simulink library "ssc_Probes_2014a_org"  (Simulink 10.0)
settings: Solver=ode45  StartTime=0.0  StopTime=10.0  RelTol=1e-3  EnableMultiTasking=on
libraries: fl_lib x50, nesl_utility x49, pe_lib x9
(part 2 of 3)

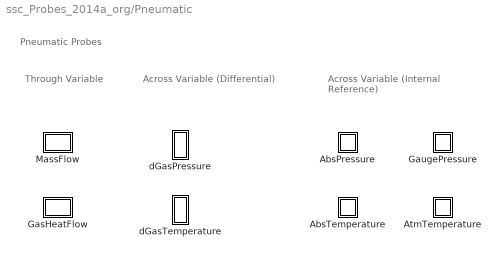
== system ssc_Probes_2014a_org/Pneumatic ==
  note: Pneumatic Probes
  note: Across Variable
      | (Internal Reference)
  note: Through
      | Variable
  note: Across Variable
      | (Differential)
  AbsPressure : Subsystem  Description=Simscape Probe  InitFcn=|
      | unit=get_param([gcb '/PS-S'],'Unit');                                              
      | set_param(gcb, 'AttributesFormatString', strcat('[', unit,']'));
      mask help: Simscape Probe
      settings: CopyFcn=|
      | if strcmp(get_param(gcb, 'LinkStatus'),'implicit') == 0;
      | set_param(gcb,'LinkStatus','inactive');
      | set_param(gcb,'LinkStatus','none');
      | end
      | set_param([gcb '/Goto'],'GotoTag', [get(gcbh,'name')]);
      | set_param([gcb '/From'],'GotoTag', [get(gcbh,'name')]);
      | h = get_param([gcb, '/PS-S'], 'PortHandles');
      | set(h.Outport(1), 'SignalNameFromLabel', [get(gcbh,'name')])
      | clear h;
      settings: NameChangeFcn=|
      | set_param([gcb '/Goto'],'GotoTag', [get(gcbh,'name')]);
      | set_param([gcb '/From'],'GotoTag', [get(gcbh,'name')]);
      | h = get_param([gcb, '/PS-S'], 'PortHandles');
      | set(h.Outport(1), 'SignalNameFromLabel', [get(gcbh,'name')])
      | clear h;
      settings: OpenFcn=|
      | if exist('logsout', 'var')
      |   vname = get(gcbh,'name');
      |   fHandle = findall(0,'Tag',vname);
      |   if isempty(fHandle)
      |   figure('Tag',vname);
      |   end;
      |   figure(findobj('Tag',vname));
      |   plot(logsout.getElement([gcb, '/PS-S'], '-blockpath').Values)
      |   title(get(gcbh,'name'));
      |   ylabel(['Pressure (' get_param([gcb '/PS-S'],'Unit') ')'] );
      | end
      mask Display: port_label('LConn', 1,'P');
  AbsTemperature : Subsystem  Description=Simscape Probe  InitFcn=|
      | unit=get_param([gcb '/PS-S'],'Unit');                                              
      | set_param(gcb, 'AttributesFormatString', strcat('[', unit,']'));
      mask help: Simscape Probe
      settings: CopyFcn=|
      | if strcmp(get_param(gcb, 'LinkStatus'),'implicit') == 0;
      | set_param(gcb,'LinkStatus','inactive');
      | set_param(gcb,'LinkStatus','none');
      | end
      | set_param([gcb '/Goto'],'GotoTag', [get(gcbh,'name')]);
      | set_param([gcb '/From'],'GotoTag', [get(gcbh,'name')]);
      | h = get_param([gcb, '/PS-S'], 'PortHandles');
      | set(h.Outport(1), 'SignalNameFromLabel', [get(gcbh,'name')])
      | clear h;
      settings: NameChangeFcn=|
      | set_param([gcb '/Goto'],'GotoTag', [get(gcbh,'name')]);
      | set_param([gcb '/From'],'GotoTag', [get(gcbh,'name')]);
      | h = get_param([gcb, '/PS-S'], 'PortHandles');
      | set(h.Outport(1), 'SignalNameFromLabel', [get(gcbh,'name')])
      | clear h;
      settings: OpenFcn=|
      | if exist('logsout', 'var')
      |   vname = get(gcbh,'name');
      |   fHandle = findall(0,'Tag',vname);
      |   if isempty(fHandle)
      |   figure('Tag',vname);
      |   end;
      |   figure(findobj('Tag',vname));
      |   plot(logsout.getElement([gcb, '/PS-S'], '-blockpath').Values)
      |   title(get(gcbh,'name'));
      |   ylabel(['Temperature (' get_param([gcb '/PS-S'],'Unit') ')'] );
      | end
      mask Display: port_label('LConn', 1,'T');
  AtmTemperature : Subsystem  Description=Simscape Probe  InitFcn=|
      | unit=get_param([gcb '/PS-S'],'Unit');                                              
      | set_param(gcb, 'AttributesFormatString', strcat('[', unit,']'));
      mask help: Simscape Probe
      settings: CopyFcn=|
      | if strcmp(get_param(gcb, 'LinkStatus'),'implicit') == 0;
      | set_param(gcb,'LinkStatus','inactive');
      | set_param(gcb,'LinkStatus','none');
      | end
      | set_param([gcb '/Goto'],'GotoTag', [get(gcbh,'name')]);
      | set_param([gcb '/From'],'GotoTag', [get(gcbh,'name')]);
      | h = get_param([gcb, '/PS-S'], 'PortHandles');
      | set(h.Outport(1), 'SignalNameFromLabel', [get(gcbh,'name')])
      | clear h;
      settings: NameChangeFcn=|
      | set_param([gcb '/Goto'],'GotoTag', [get(gcbh,'name')]);
      | set_param([gcb '/From'],'GotoTag', [get(gcbh,'name')]);
      | h = get_param([gcb, '/PS-S'], 'PortHandles');
      | set(h.Outport(1), 'SignalNameFromLabel', [get(gcbh,'name')])
      | clear h;
      settings: OpenFcn=|
      | if exist('logsout', 'var')
      |   vname = get(gcbh,'name');
      |   fHandle = findall(0,'Tag',vname);
      |   if isempty(fHandle)
      |   figure('Tag',vname);
      |   end;
      |   figure(findobj('Tag',vname));
      |   plot(logsout.getElement([gcb, '/PS-S'], '-blockpath').Values)
      |   title(get(gcbh,'name'));
      |   ylabel(['Temperature (' get_param([gcb '/PS-S'],'Unit') ')'] );
      | end
      mask Display: port_label('LConn', 1,'T');
  GasHeatFlow : Subsystem  Description=Simscape Probe  InitFcn=|
      | unit=get_param([gcb '/PS-S'],'Unit');                                              
      | set_param(gcb, 'AttributesFormatString', strcat('[', unit,']'));
      mask help: Simscape Probe
      settings: CopyFcn=|
      | if strcmp(get_param(gcb, 'LinkStatus'),'implicit') == 0;
      | set_param(gcb,'LinkStatus','inactive');
      | set_param(gcb,'LinkStatus','none');
      | end
      | set_param([gcb '/Goto'],'GotoTag', [get(gcbh,'name')]);
      | set_param([gcb '/From'],'GotoTag', [get(gcbh,'name')]);
      | h = get_param([gcb, '/PS-S'], 'PortHandles');
      | set(h.Outport(1), 'SignalNameFromLabel', [get(gcbh,'name')])
      | clear h;
      settings: NameChangeFcn=|
      | set_param([gcb '/Goto'],'GotoTag', [get(gcbh,'name')]);
      | set_param([gcb '/From'],'GotoTag', [get(gcbh,'name')]);
      | h = get_param([gcb, '/PS-S'], 'PortHandles');
      | set(h.Outport(1), 'SignalNameFromLabel', [get(gcbh,'name')])
      | clear h;
      settings: OpenFcn=|
      | if exist('logsout', 'var')
      |   vname = get(gcbh,'name');
      |   fHandle = findall(0,'Tag',vname);
      |   if isempty(fHandle)
      |   figure('Tag',vname);
      |   end;
      |   figure(findobj('Tag',vname));
      |   plot(logsout.getElement([gcb, '/PS-S'], '-blockpath').Values)
      |   title(get(gcbh,'name'));
      |   ylabel(['Heat Flow (' get_param([gcb '/PS-S'],'Unit') ')'] );
      | end
      mask Display:
      | patch([0.5 1 0.5], [0.25 .5 0.75],[0.7 0.7 0.7])
      | plot([0,0.5],[0.5,0.5]);
  GaugePressure : Subsystem  Description=Simscape Probe  InitFcn=|
      | unit=get_param([gcb '/PS-S'],'Unit');                                              
      | set_param(gcb, 'AttributesFormatString', strcat('[', unit,']'));
      mask help: Simscape Probe
      settings: CopyFcn=|
      | if strcmp(get_param(gcb, 'LinkStatus'),'implicit') == 0;
      | set_param(gcb,'LinkStatus','inactive');
      | set_param(gcb,'LinkStatus','none');
      | end
      | set_param([gcb '/Goto'],'GotoTag', [get(gcbh,'name')]);
      | set_param([gcb '/From'],'GotoTag', [get(gcbh,'name')]);
      | h = get_param([gcb, '/PS-S'], 'PortHandles');
      | set(h.Outport(1), 'SignalNameFromLabel', [get(gcbh,'name')])
      | clear h;
      settings: NameChangeFcn=|
      | set_param([gcb '/Goto'],'GotoTag', [get(gcbh,'name')]);
      | set_param([gcb '/From'],'GotoTag', [get(gcbh,'name')]);
      | h = get_param([gcb, '/PS-S'], 'PortHandles');
      | set(h.Outport(1), 'SignalNameFromLabel', [get(gcbh,'name')])
      | clear h;
      settings: OpenFcn=|
      | if exist('logsout', 'var')
      |   vname = get(gcbh,'name');
      |   fHandle = findall(0,'Tag',vname);
      |   if isempty(fHandle)
      |   figure('Tag',vname);
      |   end;
      |   figure(findobj('Tag',vname));
      |   plot(logsout.getElement([gcb, '/PS-S'], '-blockpath').Values)
      |   title(get(gcbh,'name'));
      |   ylabel(['Pressure (' get_param([gcb '/PS-S'],'Unit') ')'] );
      | end
      mask Display: port_label('LConn', 1,'P');
  MassFlow : Subsystem  Description=Simscape Probe  InitFcn=|
      | unit=get_param([gcb '/PS-S'],'Unit');                                              
      | set_param(gcb, 'AttributesFormatString', strcat('[', unit,']'));
      mask help: Simscape Probe
      settings: CopyFcn=|
      | if strcmp(get_param(gcb, 'LinkStatus'),'implicit') == 0;
      | set_param(gcb,'LinkStatus','inactive');
      | set_param(gcb,'LinkStatus','none');
      | end
      | set_param([gcb '/Goto'],'GotoTag', [get(gcbh,'name')]);
      | set_param([gcb '/From'],'GotoTag', [get(gcbh,'name')]);
      | h = get_param([gcb, '/PS-S'], 'PortHandles');
      | set(h.Outport(1), 'SignalNameFromLabel', [get(gcbh,'name')])
      | clear h;
      settings: NameChangeFcn=|
      | set_param([gcb '/Goto'],'GotoTag', [get(gcbh,'name')]);
      | set_param([gcb '/From'],'GotoTag', [get(gcbh,'name')]);
      | h = get_param([gcb, '/PS-S'], 'PortHandles');
      | set(h.Outport(1), 'SignalNameFromLabel', [get(gcbh,'name')])
      | clear h;
      settings: OpenFcn=|
      | if exist('logsout', 'var')
      |   vname = get(gcbh,'name');
      |   fHandle = findall(0,'Tag',vname);
      |   if isempty(fHandle)
      |   figure('Tag',vname);
      |   end;
      |   figure(findobj('Tag',vname));
      |   plot(logsout.getElement([gcb, '/PS-S'], '-blockpath').Values)
      |   title(get(gcbh,'name'));
      |   ylabel(['Mass Flow (' get_param([gcb '/PS-S'],'Unit') ')'] );
      | end
      mask Display:
      | patch([0.5 1 0.5], [0.25 .5 0.75],[0.7 0.7 0.7])
      | plot([0,0.5],[0.5,0.5]);
  dGasPressure : Subsystem  Description=Simscape Probe  InitFcn=|
      | unit=get_param([gcb '/PS-S'],'Unit');                                              
      | set_param(gcb, 'AttributesFormatString', strcat('[', unit,']'));
      mask help: Simscape Probe
      settings: CopyFcn=|
      | if strcmp(get_param(gcb, 'LinkStatus'),'implicit') == 0;
      | set_param(gcb,'LinkStatus','inactive');
      | set_param(gcb,'LinkStatus','none');
      | end
      | set_param([gcb '/Goto'],'GotoTag', [get(gcbh,'name')]);
      | set_param([gcb '/From'],'GotoTag', [get(gcbh,'name')]);
      | h = get_param([gcb, '/PS-S'], 'PortHandles');
      | set(h.Outport(1), 'SignalNameFromLabel', [get(gcbh,'name')])
      | clear h;
      settings: NameChangeFcn=|
      | set_param([gcb '/Goto'],'GotoTag', [get(gcbh,'name')]);
      | set_param([gcb '/From'],'GotoTag', [get(gcbh,'name')]);
      | h = get_param([gcb, '/PS-S'], 'PortHandles');
      | set(h.Outport(1), 'SignalNameFromLabel', [get(gcbh,'name')])
      | clear h;
      settings: OpenFcn=|
      | if exist('logsout', 'var')
      |   vname = get(gcbh,'name');
      |   fHandle = findall(0,'Tag',vname);
      |   if isempty(fHandle)
      |   figure('Tag',vname);
      |   end;
      |   figure(findobj('Tag',vname));
      |   plot(logsout.getElement([gcb, '/PS-S'], '-blockpath').Values)
      |   title(get(gcbh,'name'));
      |   ylabel(['Pressure (' get_param([gcb '/PS-S'],'Unit') ')'] );
      | end
      mask Display:
      | port_label('RConn', 1,'-');
      | port_label('LConn', 1,'+');
  dGasTemperature : Subsystem  Description=Simscape Probe  InitFcn=|
      | unit=get_param([gcb '/PS-S'],'Unit');                                              
      | set_param(gcb, 'AttributesFormatString', strcat('[', unit,']'));
      mask help: Simscape Probe
      settings: CopyFcn=|
      | if strcmp(get_param(gcb, 'LinkStatus'),'implicit') == 0;
      | set_param(gcb,'LinkStatus','inactive');
      | set_param(gcb,'LinkStatus','none');
      | end
      | set_param([gcb '/Goto'],'GotoTag', [get(gcbh,'name')]);
      | set_param([gcb '/From'],'GotoTag', [get(gcbh,'name')]);
      | h = get_param([gcb, '/PS-S'], 'PortHandles');
      | set(h.Outport(1), 'SignalNameFromLabel', [get(gcbh,'name')])
      | clear h;
      settings: NameChangeFcn=|
      | set_param([gcb '/Goto'],'GotoTag', [get(gcbh,'name')]);
      | set_param([gcb '/From'],'GotoTag', [get(gcbh,'name')]);
      | h = get_param([gcb, '/PS-S'], 'PortHandles');
      | set(h.Outport(1), 'SignalNameFromLabel', [get(gcbh,'name')])
      | clear h;
      settings: OpenFcn=|
      | if exist('logsout', 'var')
      |   vname = get(gcbh,'name');
      |   fHandle = findall(0,'Tag',vname);
      |   if isempty(fHandle)
      |   figure('Tag',vname);
      |   end;
      |   figure(findobj('Tag',vname));
      |   plot(logsout.getElement([gcb, '/PS-S'], '-blockpath').Values)
      |   title(get(gcbh,'name'));
      |   ylabel(['Temperature (' get_param([gcb '/PS-S'],'Unit') ')'] );
      | end
      mask Display:
      | port_label('RConn', 1,'-');
      | port_label('LConn', 1,'+');

== system ssc_Probes_2014a_org/Thermal ==
  note: Thermal Probes
  note: Across Variable
      | (Internal Reference)
  note: Through
      | Variable
  note: Across Variable
      | (Differential)
  HeatFlow : Subsystem  Description=Simscape Probe  InitFcn=|
      | unit=get_param([gcb '/PS-S'],'Unit');                                              
      | set_param(gcb, 'AttributesFormatString', strcat('[', unit,']'));
      mask help: Simscape Probe
      settings: CopyFcn=|
      | if strcmp(get_param(gcb, 'LinkStatus'),'implicit') == 0;
      | set_param(gcb,'LinkStatus','inactive');
      | set_param(gcb,'LinkStatus','none');
      | end
      | set_param([gcb '/Goto'],'GotoTag', [get(gcbh,'name')]);
      | set_param([gcb '/From'],'GotoTag', [get(gcbh,'name')]);
      | h = get_param([gcb, '/PS-S'], 'PortHandles');
      | set(h.Outport(1), 'SignalNameFromLabel', [get(gcbh,'name')])
      | clear h;
      settings: NameChangeFcn=|
      | set_param([gcb '/Goto'],'GotoTag', [get(gcbh,'name')]);
      | set_param([gcb '/From'],'GotoTag', [get(gcbh,'name')]);
      | h = get_param([gcb, '/PS-S'], 'PortHandles');
      | set(h.Outport(1), 'SignalNameFromLabel', [get(gcbh,'name')])
      | clear h;
      settings: OpenFcn=|
      | if exist('logsout', 'var')
      |   vname = get(gcbh,'name');
      |   fHandle = findall(0,'Tag',vname);
      |   if isempty(fHandle)
      |   figure('Tag',vname);
      |   end;
      |   figure(findobj('Tag',vname));
      |   plot(logsout.getElement([gcb, '/PS-S'], '-blockpath').Values)
      |   title(get(gcbh,'name'));
      |   ylabel(['Heat Flow (' get_param([gcb '/PS-S'],'Unit') ')'] );
      | end
      mask Display:
      | patch([0.5 1 0.5], [0.25 .5 0.75],[0.7 0.7 0.7])
      | plot([0,0.5],[0.5,0.5]);
  Temperature : Subsystem  Description=Simscape Probe  InitFcn=|
      | unit=get_param([gcb '/PS-S'],'Unit');                                              
      | set_param(gcb, 'AttributesFormatString', strcat('[', unit,']'));
      mask help: Simscape Probe
      settings: CopyFcn=|
      | if strcmp(get_param(gcb, 'LinkStatus'),'implicit') == 0;
      | set_param(gcb,'LinkStatus','inactive');
      | set_param(gcb,'LinkStatus','none');
      | end
      | set_param([gcb '/Goto'],'GotoTag', [get(gcbh,'name')]);
      | set_param([gcb '/From'],'GotoTag', [get(gcbh,'name')]);
      | h = get_param([gcb, '/PS-S'], 'PortHandles');
      | set(h.Outport(1), 'SignalNameFromLabel', [get(gcbh,'name')])
      | clear h;
      settings: NameChangeFcn=|
      | set_param([gcb '/Goto'],'GotoTag', [get(gcbh,'name')]);
      | set_param([gcb '/From'],'GotoTag', [get(gcbh,'name')]);
      | h = get_param([gcb, '/PS-S'], 'PortHandles');
      | set(h.Outport(1), 'SignalNameFromLabel', [get(gcbh,'name')])
      | clear h;
      settings: OpenFcn=|
      | if exist('logsout', 'var')
      |   vname = get(gcbh,'name');
      |   fHandle = findall(0,'Tag',vname);
      |   if isempty(fHandle)
      |   figure('Tag',vname);
      |   end;
      |   figure(findobj('Tag',vname));
      |   plot(logsout.getElement([gcb, '/PS-S'], '-blockpath').Values)
      |   title(get(gcbh,'name'));
      |   ylabel(['Temperature (' get_param([gcb '/PS-S'],'Unit') ')'] );
      | end
      mask Display: port_label('LConn', 1,'T');
  dTemperature : Subsystem  Description=Simscape Probe  InitFcn=|
      | unit=get_param([gcb '/PS-S'],'Unit');                                              
      | set_param(gcb, 'AttributesFormatString', strcat('[', unit,']'));
      mask help: Simscape Probe
      settings: CopyFcn=|
      | if strcmp(get_param(gcb, 'LinkStatus'),'implicit') == 0;
      | set_param(gcb,'LinkStatus','inactive');
      | set_param(gcb,'LinkStatus','none');
      | end
      | set_param([gcb '/Goto'],'GotoTag', [get(gcbh,'name')]);
      | set_param([gcb '/From'],'GotoTag', [get(gcbh,'name')]);
      | h = get_param([gcb, '/PS-S'], 'PortHandles');
      | set(h.Outport(1), 'SignalNameFromLabel', [get(gcbh,'name')])
      | clear h;
      settings: NameChangeFcn=|
      | set_param([gcb '/Goto'],'GotoTag', [get(gcbh,'name')]);
      | set_param([gcb '/From'],'GotoTag', [get(gcbh,'name')]);
      | h = get_param([gcb, '/PS-S'], 'PortHandles');
      | set(h.Outport(1), 'SignalNameFromLabel', [get(gcbh,'name')])
      | clear h;
      settings: OpenFcn=|
      | if exist('logsout', 'var')
      |   vname = get(gcbh,'name');
      |   fHandle = findall(0,'Tag',vname);
      |   if isempty(fHandle)
      |   figure('Tag',vname);
      |   end;
      |   figure(findobj('Tag',vname));
      |   plot(logsout.getElement([gcb, '/PS-S'], '-blockpath').Values)
      |   title(get(gcbh,'name'));
      |   ylabel(['Temperature (' get_param([gcb '/PS-S'],'Unit') ')'] );
      | end
      mask Display:
      | port_label('RConn', 1,'-');
      | port_label('LConn', 1,'+');

== system ssc_Probes_2014a_org/ThermalLiquid ==
  note: Across Variable
      | (Differential)
  note: Through
      | Variable
  note: Across Variable
      | (Internal Reference)
  note: Thermal Probes
  AbsPressure_TL : Subsystem  Description=Simscape Probe  InitFcn=|
      | unit=get_param([gcb '/PS-S'],'Unit');                                              
      | set_param(gcb, 'AttributesFormatString', strcat('[', unit,']'));
      mask help: Simscape Probe
      settings: CopyFcn=|
      | if strcmp(get_param(gcb, 'LinkStatus'),'implicit') == 0;
      | set_param(gcb,'LinkStatus','inactive');
      | set_param(gcb,'LinkStatus','none');
      | end
      | set_param([gcb '/Goto'],'GotoTag', [get(gcbh,'name')]);
      | set_param([gcb '/From'],'GotoTag', [get(gcbh,'name')]);
      | h = get_param([gcb, '/PS-S'], 'PortHandles');
      | set(h.Outport(1), 'SignalNameFromLabel', [get(gcbh,'name')])
      | clear h;
      settings: NameChangeFcn=|
      | set_param([gcb '/Goto'],'GotoTag', [get(gcbh,'name')]);
      | set_param([gcb '/From'],'GotoTag', [get(gcbh,'name')]);
      | h = get_param([gcb, '/PS-S'], 'PortHandles');
      | set(h.Outport(1), 'SignalNameFromLabel', [get(gcbh,'name')])
      | clear h;
      settings: OpenFcn=|
      | if exist('logsout', 'var')
      |   vname = get(gcbh,'name');
      |   fHandle = findall(0,'Tag',vname);
      |   if isempty(fHandle)
      |   figure('Tag',vname);
      |   end;
      |   figure(findobj('Tag',vname));
      |   plot(logsout.getElement([gcb, '/PS-S'], '-blockpath').Values)
      |   title(get(gcbh,'name'));
      |   ylabel(['Pressure (' get_param([gcb '/PS-S'],'Unit') ')'] );
      | end
      mask Display: port_label('LConn', 1,'P');
  AbsTemperature_TL : Subsystem  Description=Simscape Probe  InitFcn=|
      | unit=get_param([gcb '/PS-S'],'Unit');                                              
      | set_param(gcb, 'AttributesFormatString', strcat('[', unit,']'));
      mask help: Simscape Probe
      settings: CopyFcn=|
      | if strcmp(get_param(gcb, 'LinkStatus'),'implicit') == 0;
      | set_param(gcb,'LinkStatus','inactive');
      | set_param(gcb,'LinkStatus','none');
      | end
      | set_param([gcb '/Goto'],'GotoTag', [get(gcbh,'name')]);
      | set_param([gcb '/From'],'GotoTag', [get(gcbh,'name')]);
      | h = get_param([gcb, '/PS-S'], 'PortHandles');
      | set(h.Outport(1), 'SignalNameFromLabel', [get(gcbh,'name')])
      | clear h;
      settings: NameChangeFcn=|
      | set_param([gcb '/Goto'],'GotoTag', [get(gcbh,'name')]);
      | set_param([gcb '/From'],'GotoTag', [get(gcbh,'name')]);
      | h = get_param([gcb, '/PS-S'], 'PortHandles');
      | set(h.Outport(1), 'SignalNameFromLabel', [get(gcbh,'name')])
      | clear h;
      settings: OpenFcn=|
      | if exist('logsout', 'var')
      |   vname = get(gcbh,'name');
      |   fHandle = findall(0,'Tag',vname);
      |   if isempty(fHandle)
      |   figure('Tag',vname);
      |   end;
      |   figure(findobj('Tag',vname));
      |   plot(logsout.getElement([gcb, '/PS-S'], '-blockpath').Values)
      |   title(get(gcbh,'name'));
      |   ylabel(['Temperature (' get_param([gcb '/PS-S'],'Unit') ')'] );
      | end
      mask Display: port_label('LConn', 1,'T');
  MassFlow_TL : Subsystem  Description=Simscape Probe  InitFcn=|
      | unit=get_param([gcb '/PS-S'],'Unit');                                              
      | set_param(gcb, 'AttributesFormatString', strcat('[', unit,']'));
      mask help: Simscape Probe
      settings: CopyFcn=|
      | if strcmp(get_param(gcb, 'LinkStatus'),'implicit') == 0;
      | set_param(gcb,'LinkStatus','inactive');
      | set_param(gcb,'LinkStatus','none');
      | end
      | set_param([gcb '/Goto'],'GotoTag', [get(gcbh,'name')]);
      | set_param([gcb '/From'],'GotoTag', [get(gcbh,'name')]);
      | h = get_param([gcb, '/PS-S'], 'PortHandles');
      | set(h.Outport(1), 'SignalNameFromLabel', [get(gcbh,'name')])
      | clear h;
      settings: NameChangeFcn=|
      | set_param([gcb '/Goto'],'GotoTag', [get(gcbh,'name')]);
      | set_param([gcb '/From'],'GotoTag', [get(gcbh,'name')]);
      | h = get_param([gcb, '/PS-S'], 'PortHandles');
      | set(h.Outport(1), 'SignalNameFromLabel', [get(gcbh,'name')])
      | clear h;
      settings: OpenFcn=|
      | if exist('logsout', 'var')
      |   vname = get(gcbh,'name');
      |   fHandle = findall(0,'Tag',vname);
      |   if isempty(fHandle)
      |   figure('Tag',vname);
      |   end;
      |   figure(findobj('Tag',vname));
      |   plot(logsout.getElement([gcb, '/PS-S'], '-blockpath').Values)
      |   title(get(gcbh,'name'));
      |   ylabel(['Mass Flow (' get_param([gcb '/PS-S'],'Unit') ')'] );
      | end
      mask Display:
      | patch([0.5 1 0.5], [0.25 .5 0.75],[0.7 0.7 0.7])
      | plot([0,0.5],[0.5,0.5]);
  ThermalFlux_TL : Subsystem  Description=Simscape Probe  InitFcn=|
      | unit=get_param([gcb '/PS-S'],'Unit');                                              
      | set_param(gcb, 'AttributesFormatString', strcat('[', unit,']'));
      mask help: Simscape Probe
      settings: CopyFcn=|
      | if strcmp(get_param(gcb, 'LinkStatus'),'implicit') == 0;
      | set_param(gcb,'LinkStatus','inactive');
      | set_param(gcb,'LinkStatus','none');
      | end
      | set_param([gcb '/Goto'],'GotoTag', [get(gcbh,'name')]);
      | set_param([gcb '/From'],'GotoTag', [get(gcbh,'name')]);
      | h = get_param([gcb, '/PS-S'], 'PortHandles');
      | set(h.Outport(1), 'SignalNameFromLabel', [get(gcbh,'name')])
      | clear h;
      settings: NameChangeFcn=|
      | set_param([gcb '/Goto'],'GotoTag', [get(gcbh,'name')]);
      | set_param([gcb '/From'],'GotoTag', [get(gcbh,'name')]);
      | h = get_param([gcb, '/PS-S'], 'PortHandles');
      | set(h.Outport(1), 'SignalNameFromLabel', [get(gcbh,'name')])
      | clear h;
      settings: OpenFcn=|
      | if exist('logsout', 'var')
      |   vname = get(gcbh,'name');
      |   fHandle = findall(0,'Tag',vname);
      |   if isempty(fHandle)
      |   figure('Tag',vname);
      |   end;
      |   figure(findobj('Tag',vname));
      |   plot(logsout.getElement([gcb, '/PS-S'], '-blockpath').Values)
      |   title(get(gcbh,'name'));
      |   ylabel(['Thermal Flux (' get_param([gcb '/PS-S'],'Unit') ')'] );
      | end
      mask Display:
      | patch([0.5 1 0.5], [0.25 .5 0.75],[0.7 0.7 0.7])
      | plot([0,0.5],[0.5,0.5]);
  dPressure_TL : Subsystem  Description=Simscape Probe  InitFcn=|
      | unit=get_param([gcb '/PS-S'],'Unit');                                              
      | set_param(gcb, 'AttributesFormatString', strcat('[', unit,']'));
      mask help: Simscape Probe
      settings: CopyFcn=|
      | if strcmp(get_param(gcb, 'LinkStatus'),'implicit') == 0;
      | set_param(gcb,'LinkStatus','inactive');
      | set_param(gcb,'LinkStatus','none');
      | end
      | set_param([gcb '/Goto'],'GotoTag', [get(gcbh,'name')]);
      | set_param([gcb '/From'],'GotoTag', [get(gcbh,'name')]);
      | h = get_param([gcb, '/PS-S'], 'PortHandles');
      | set(h.Outport(1), 'SignalNameFromLabel', [get(gcbh,'name')])
      | clear h;
      settings: NameChangeFcn=|
      | set_param([gcb '/Goto'],'GotoTag', [get(gcbh,'name')]);
      | set_param([gcb '/From'],'GotoTag', [get(gcbh,'name')]);
      | h = get_param([gcb, '/PS-S'], 'PortHandles');
      | set(h.Outport(1), 'SignalNameFromLabel', [get(gcbh,'name')])
      | clear h;
      settings: OpenFcn=|
      | if exist('logsout', 'var')
      |   vname = get(gcbh,'name');
      |   fHandle = findall(0,'Tag',vname);
      |   if isempty(fHandle)
      |   figure('Tag',vname);
      |   end;
      |   figure(findobj('Tag',vname));
      |   plot(logsout.getElement([gcb, '/PS-S'], '-blockpath').Values)
      |   title(get(gcbh,'name'));
      |   ylabel(['Pressure (' get_param([gcb '/PS-S'],'Unit') ')'] );
      | end
      mask Display:
      | port_label('RConn', 1,'-');
      | port_label('LConn', 1,'+');
  dTemperature_TL : Subsystem  Description=Simscape Probe  InitFcn=|
      | unit=get_param([gcb '/PS-S'],'Unit');                                              
      | set_param(gcb, 'AttributesFormatString', strcat('[', unit,']'));
      mask help: Simscape Probe
      settings: CopyFcn=|
      | if strcmp(get_param(gcb, 'LinkStatus'),'implicit') == 0;
      | set_param(gcb,'LinkStatus','inactive');
      | set_param(gcb,'LinkStatus','none');
      | end
      | set_param([gcb '/Goto'],'GotoTag', [get(gcbh,'name')]);
      | set_param([gcb '/From'],'GotoTag', [get(gcbh,'name')]);
      | h = get_param([gcb, '/PS-S'], 'PortHandles');
      | set(h.Outport(1), 'SignalNameFromLabel', [get(gcbh,'name')])
      | clear h;
      settings: NameChangeFcn=|
      | set_param([gcb '/Goto'],'GotoTag', [get(gcbh,'name')]);
      | set_param([gcb '/From'],'GotoTag', [get(gcbh,'name')]);
      | h = get_param([gcb, '/PS-S'], 'PortHandles');
      | set(h.Outport(1), 'SignalNameFromLabel', [get(gcbh,'name')])
      | clear h;
      settings: OpenFcn=|
      | if exist('logsout', 'var')
      |   vname = get(gcbh,'name');
      |   fHandle = findall(0,'Tag',vname);
      |   if isempty(fHandle)
      |   figure('Tag',vname);
      |   end;
      |   figure(findobj('Tag',vname));
      |   plot(logsout.getElement([gcb, '/PS-S'], '-blockpath').Values)
      |   title(get(gcbh,'name'));
      |   ylabel(['Temperature (' get_param([gcb '/PS-S'],'Unit') ')'] );
      | end
      mask Display:
      | port_label('RConn', 1,'-');
      | port_label('LConn', 1,'+');

== system ssc_Probes_2014a_org/DocBlock/EmptySubsystem ==

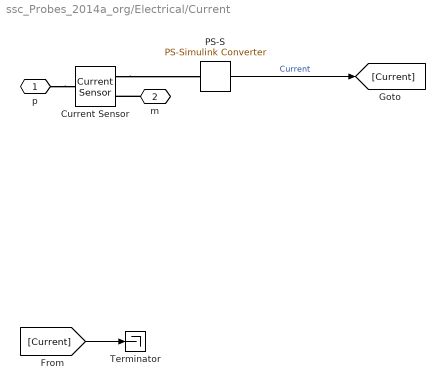
== system ssc_Probes_2014a_org/Electrical/Current ==
  Current Sensor : fl_lib/Electrical/Electrical Sensors/Current Sensor
  PS-S : nesl_utility/PS-Simulink Converter  PhysicalDomain=network_engine_domain  SubClassName=ps_output  LeftPortType=input  RightPortType=output  PseudoPeriodic=off  Frequencies=[]  Unit=A  AffineConversion=off
  Terminator : Terminator
  p : PMIOPort  Side=Left
  m : PMIOPort  Port=2  Side=Right
  wires:
  PS-S/1 -> [Current]  "Current"
  [Current] -> Terminator/1
  connections:
  m/RConn1 -- Current Sensor/RConn2
  p/RConn1 -- Current Sensor/LConn1
  Current Sensor/RConn1 -- PS-S/LConn1

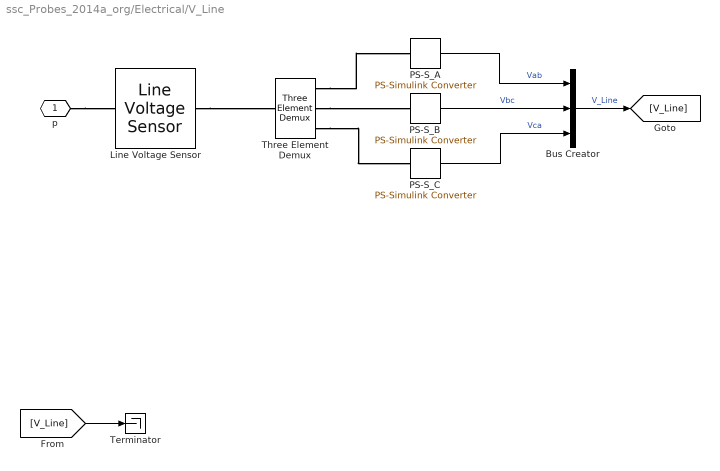
== system ssc_Probes_2014a_org/Electrical/V_Line ==
  Bus Creator : BusCreator  Inputs=3
  Line Voltage Sensor : pe_lib/Sensors/Line Voltage Sensor
      settings: SourceProductName=Simscape Electrical  SourceProductBaseCode=PS
  PS-S_A : nesl_utility/PS-Simulink Converter  PhysicalDomain=network_engine_domain  SubClassName=ps_output  LeftPortType=input  RightPortType=output  PseudoPeriodic=off  Frequencies=[]  Unit=V  AffineConversion=off
  PS-S_B : nesl_utility/PS-Simulink Converter  PhysicalDomain=network_engine_domain  SubClassName=ps_output  LeftPortType=input  RightPortType=output  PseudoPeriodic=off  Frequencies=[]  Unit=V  AffineConversion=off
  PS-S_C : nesl_utility/PS-Simulink Converter  PhysicalDomain=network_engine_domain  SubClassName=ps_output  LeftPortType=input  RightPortType=output  PseudoPeriodic=off  Frequencies=[]  Unit=V  AffineConversion=off
  Terminator : Terminator
  Three Element Demux : pe_lib/Sensors/Three Element Demux  LocalVarLogging=[]
      settings: SourceProductName=Simscape Electrical  SourceProductBaseCode=PS
  p : PMIOPort  Side=Left
  wires:
  Bus Creator/1 -> [V_Line]  "V_Line"
  PS-S_C/1 -> Bus Creator/3  "Vca"
  PS-S_B/1 -> Bus Creator/2  "Vbc"
  PS-S_A/1 -> Bus Creator/1  "Vab"
  [V_Line] -> Terminator/1
  connections:
  Line Voltage Sensor/RConn1 -- Three Element Demux/LConn1
  Three Element Demux/RConn2 -- PS-S_B/LConn1
  Three Element Demux/RConn1 -- PS-S_A/LConn1
  Three Element Demux/RConn3 -- PS-S_C/LConn1
  p/RConn1 -- Line Voltage Sensor/LConn1

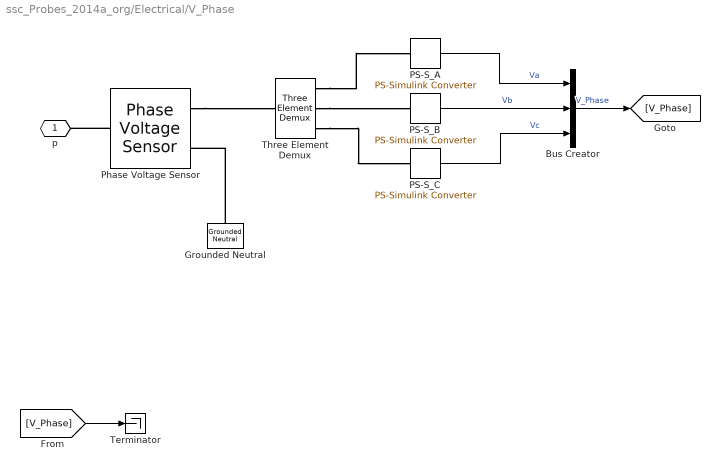
== system ssc_Probes_2014a_org/Electrical/V_Phase ==
  Bus Creator : BusCreator  Inputs=3
  Grounded Neutral : pe_lib/Connections/Grounded Neutral  LocalVarNames=|i_a|i_b|i_c  LocalVarDescs=|i_a|i_b|i_c  LocalVarLogging=[0 0 0]  i_a_Log=off  i_b_Log=off  i_c_Log=off
      settings: SourceProductName=Simscape Electrical  SourceProductBaseCode=PS
  PS-S_A : nesl_utility/PS-Simulink Converter  PhysicalDomain=network_engine_domain  SubClassName=ps_output  LeftPortType=input  RightPortType=output  PseudoPeriodic=off  Frequencies=[]  Unit=V  AffineConversion=off
  PS-S_B : nesl_utility/PS-Simulink Converter  PhysicalDomain=network_engine_domain  SubClassName=ps_output  LeftPortType=input  RightPortType=output  PseudoPeriodic=off  Frequencies=[]  Unit=V  AffineConversion=off
  PS-S_C : nesl_utility/PS-Simulink Converter  PhysicalDomain=network_engine_domain  SubClassName=ps_output  LeftPortType=input  RightPortType=output  PseudoPeriodic=off  Frequencies=[]  Unit=V  AffineConversion=off
  Phase Voltage Sensor : pe_lib/Sensors/Phase Voltage Sensor
      settings: SourceProductName=Simscape Electrical  SourceProductBaseCode=PS
  Terminator : Terminator
  Three Element Demux : pe_lib/Sensors/Three Element Demux  LocalVarLogging=[]
      settings: SourceProductName=Simscape Electrical  SourceProductBaseCode=PS
  p : PMIOPort  Side=Left
  wires:
  [V_Phase] -> Terminator/1
  PS-S_A/1 -> Bus Creator/1  "Va"
  PS-S_B/1 -> Bus Creator/2  "Vb"
  PS-S_C/1 -> Bus Creator/3  "Vc"
  Bus Creator/1 -> [V_Phase]  "V_Phase"
  connections:
  Phase Voltage Sensor/LConn1 -- p/RConn1
  Three Element Demux/RConn3 -- PS-S_C/LConn1
  Three Element Demux/RConn1 -- PS-S_A/LConn1
  Three Element Demux/RConn2 -- PS-S_B/LConn1
  Phase Voltage Sensor/RConn1 -- Three Element Demux/LConn1
  Grounded Neutral/LConn1 -- Phase Voltage Sensor/RConn2

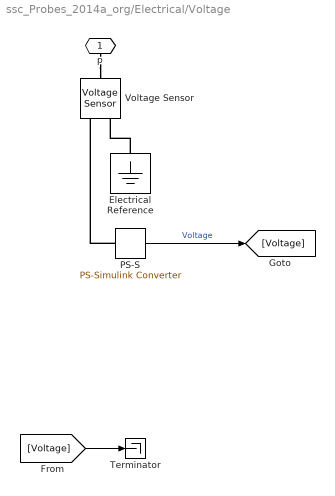
== system ssc_Probes_2014a_org/Electrical/Voltage ==
  Electrical Reference : fl_lib/Electrical/Electrical Elements/Electrical Reference  i_Log=off  LocalVarNames=|i  LocalVarDescs=|i  LocalVarLogging=0
  PS-S : nesl_utility/PS-Simulink Converter  PhysicalDomain=network_engine_domain  SubClassName=ps_output  LeftPortType=input  RightPortType=output  PseudoPeriodic=off  Frequencies=[]  Unit=V  AffineConversion=off
  Terminator : Terminator
  Voltage Sensor : fl_lib/Electrical/Electrical Sensors/Voltage Sensor
  p : PMIOPort  Side=Left
  wires:
  PS-S/1 -> [Voltage]  "Voltage"
  [Voltage] -> Terminator/1
  connections:
  Electrical Reference/LConn1 -- Voltage Sensor/RConn2
  PS-S/LConn1 -- Voltage Sensor/RConn1
  p/RConn1 -- Voltage Sensor/LConn1

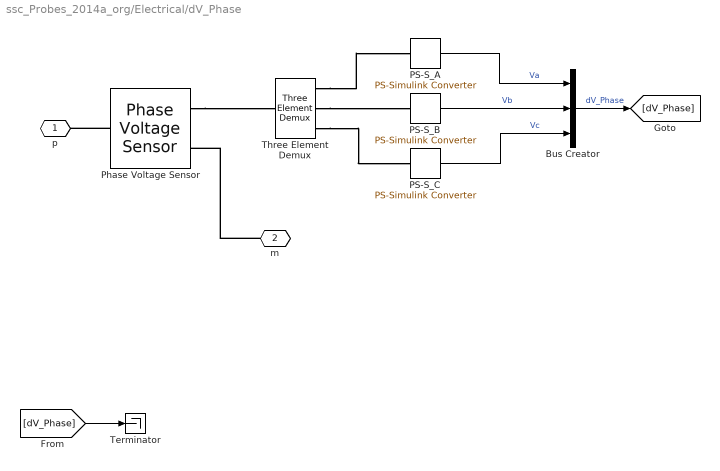
== system ssc_Probes_2014a_org/Electrical/dV_Phase ==
  Bus Creator : BusCreator  Inputs=3
  PS-S_A : nesl_utility/PS-Simulink Converter  PhysicalDomain=network_engine_domain  SubClassName=ps_output  LeftPortType=input  RightPortType=output  PseudoPeriodic=off  Frequencies=[]  Unit=V  AffineConversion=off
  PS-S_B : nesl_utility/PS-Simulink Converter  PhysicalDomain=network_engine_domain  SubClassName=ps_output  LeftPortType=input  RightPortType=output  PseudoPeriodic=off  Frequencies=[]  Unit=V  AffineConversion=off
  PS-S_C : nesl_utility/PS-Simulink Converter  PhysicalDomain=network_engine_domain  SubClassName=ps_output  LeftPortType=input  RightPortType=output  PseudoPeriodic=off  Frequencies=[]  Unit=V  AffineConversion=off
  Phase Voltage Sensor : pe_lib/Sensors/Phase Voltage Sensor
      settings: SourceProductName=Simscape Electrical  SourceProductBaseCode=PS
  Terminator : Terminator
  Three Element Demux : pe_lib/Sensors/Three Element Demux  LocalVarLogging=[]
      settings: SourceProductName=Simscape Electrical  SourceProductBaseCode=PS
  p : PMIOPort  Side=Left
  m : PMIOPort  Port=2  Side=Right
  wires:
  Bus Creator/1 -> [dV_Phase]  "dV_Phase"
  PS-S_C/1 -> Bus Creator/3  "Vc"
  PS-S_B/1 -> Bus Creator/2  "Vb"
  PS-S_A/1 -> Bus Creator/1  "Va"
  [dV_Phase] -> Terminator/1
  connections:
  m/RConn1 -- Phase Voltage Sensor/RConn2
  Phase Voltage Sensor/RConn1 -- Three Element Demux/LConn1
  Three Element Demux/RConn2 -- PS-S_B/LConn1
  Three Element Demux/RConn1 -- PS-S_A/LConn1
  Three Element Demux/RConn3 -- PS-S_C/LConn1
  Phase Voltage Sensor/LConn1 -- p/RConn1

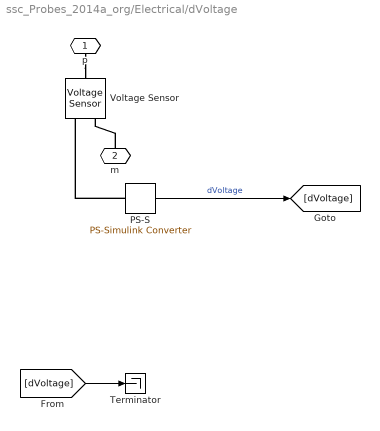
== system ssc_Probes_2014a_org/Electrical/dVoltage ==
  PS-S : nesl_utility/PS-Simulink Converter  PhysicalDomain=network_engine_domain  SubClassName=ps_output  LeftPortType=input  RightPortType=output  PseudoPeriodic=off  Frequencies=[]  Unit=V  AffineConversion=off
  Terminator : Terminator
  Voltage Sensor : fl_lib/Electrical/Electrical Sensors/Voltage Sensor
  p : PMIOPort  Side=Left
  m : PMIOPort  Port=2  Side=Right
  wires:
  PS-S/1 -> [dVoltage]  "dVoltage"
  [dVoltage] -> Terminator/1
  connections:
  p/RConn1 -- Voltage Sensor/LConn1
  PS-S/LConn1 -- Voltage Sensor/RConn1
  m/RConn1 -- Voltage Sensor/RConn2

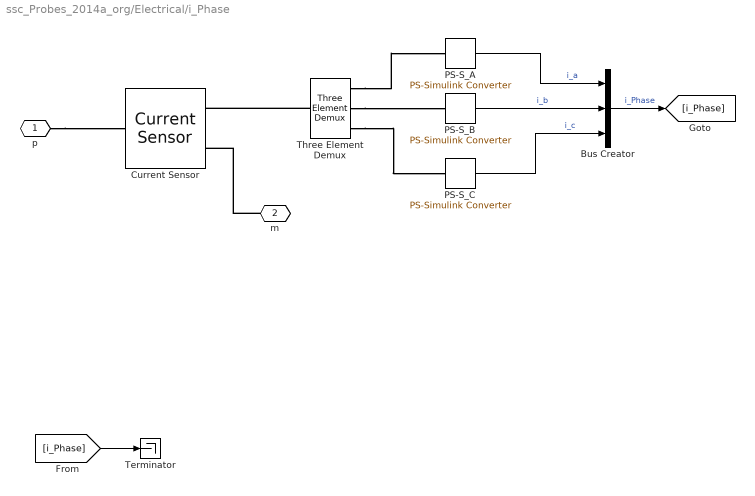
== system ssc_Probes_2014a_org/Electrical/i_Phase ==
  Bus Creator : BusCreator  Inputs=3
  Current Sensor : pe_lib/Sensors/Current Sensor
      settings: SourceProductName=Simscape Electrical  SourceProductBaseCode=PS
  PS-S_A : nesl_utility/PS-Simulink Converter  PhysicalDomain=network_engine_domain  SubClassName=ps_output  LeftPortType=input  RightPortType=output  PseudoPeriodic=off  Frequencies=[]  Unit=A  AffineConversion=off
  PS-S_B : nesl_utility/PS-Simulink Converter  PhysicalDomain=network_engine_domain  SubClassName=ps_output  LeftPortType=input  RightPortType=output  PseudoPeriodic=off  Frequencies=[]  Unit=A  AffineConversion=off
  PS-S_C : nesl_utility/PS-Simulink Converter  PhysicalDomain=network_engine_domain  SubClassName=ps_output  LeftPortType=input  RightPortType=output  PseudoPeriodic=off  Frequencies=[]  Unit=A  AffineConversion=off
  Terminator : Terminator
  Three Element Demux : pe_lib/Sensors/Three Element Demux  LocalVarLogging=[]
      settings: SourceProductName=Simscape Electrical  SourceProductBaseCode=PS
  p : PMIOPort  Side=Left
  m : PMIOPort  Port=2  Side=Right
  wires:
  [i_Phase] -> Terminator/1
  PS-S_A/1 -> Bus Creator/1  "i_a"
  PS-S_B/1 -> Bus Creator/2  "i_b"
  PS-S_C/1 -> Bus Creator/3  "i_c"
  Bus Creator/1 -> [i_Phase]  "i_Phase"
  connections:
  m/RConn1 -- Current Sensor/RConn2
  p/RConn1 -- Current Sensor/LConn1
  Three Element Demux/RConn3 -- PS-S_C/LConn1
  Three Element Demux/RConn2 -- PS-S_B/LConn1
  Three Element Demux/RConn1 -- PS-S_A/LConn1
  Three Element Demux/LConn1 -- Current Sensor/RConn1

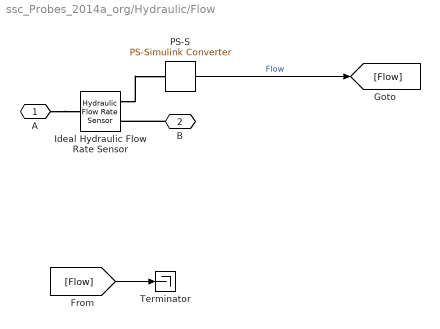
== system ssc_Probes_2014a_org/Hydraulic/Flow ==
  Ideal Hydraulic Flow Rate Sensor : fl_lib/Hydraulic/Hydraulic Sensors/Hydraulic Flow Rate Sensor
      settings: SourceProductName=Simscape
  PS-S : nesl_utility/PS-Simulink Converter  PhysicalDomain=network_engine_domain  SubClassName=ps_output  LeftPortType=input  RightPortType=output  PseudoPeriodic=off  Frequencies=[]  Unit=m^3/s  AffineConversion=off
  Terminator : Terminator
  A : PMIOPort  Side=Left
  B : PMIOPort  Port=2  Side=Right
  wires:
  PS-S/1 -> [Flow]  "Flow"
  [Flow] -> Terminator/1
  connections:
  B/RConn1 -- Ideal Hydraulic Flow Rate Sensor/RConn2
  Ideal Hydraulic Flow Rate Sensor/RConn1 -- PS-S/LConn1
  A/RConn1 -- Ideal Hydraulic Flow Rate Sensor/LConn1

== system ssc_Probes_2014a_org/Hydraulic/Pressure ==
  Hydraulic Reference : fl_lib/Hydraulic/Hydraulic Elements/Hydraulic Reference  q_Log=off  LocalVarNames=|q  LocalVarDescs=|q  LocalVarLogging=0
      settings: SourceProductName=Simscape
  Ideal Hydraulic Pressure Sensor : fl_lib/Hydraulic/Hydraulic Sensors/Hydraulic Pressure Sensor
      settings: SourceProductName=Simscape
  PS-S : nesl_utility/PS-Simulink Converter  PhysicalDomain=network_engine_domain  SubClassName=ps_output  LeftPortType=input  RightPortType=output  PseudoPeriodic=off  Frequencies=[]  Unit=Pa  AffineConversion=off
  Terminator : Terminator
  A : PMIOPort  Side=Left
  wires:
  PS-S/1 -> [Pressure]  "Pressure"
  [Pressure] -> Terminator/1
  connections:
  PS-S/LConn1 -- Ideal Hydraulic Pressure Sensor/RConn2
  Hydraulic Reference/LConn1 -- Ideal Hydraulic Pressure Sensor/RConn1
  A/RConn1 -- Ideal Hydraulic Pressure Sensor/LConn1

== system ssc_Probes_2014a_org/Hydraulic/dPressure ==
  Ideal Hydraulic Pressure Sensor : fl_lib/Hydraulic/Hydraulic Sensors/Hydraulic Pressure Sensor
      settings: SourceProductName=Simscape
  PS-S : nesl_utility/PS-Simulink Converter  PhysicalDomain=network_engine_domain  SubClassName=ps_output  LeftPortType=input  RightPortType=output  PseudoPeriodic=off  Frequencies=[]  Unit=Pa  AffineConversion=off
  Terminator : Terminator
  A : PMIOPort  Side=Left
  B : PMIOPort  Port=2  Side=Right
  wires:
  PS-S/1 -> [dPressure]  "dPressure"
  [dPressure] -> Terminator/1
  connections:
  A/RConn1 -- Ideal Hydraulic Pressure Sensor/LConn1
  B/RConn1 -- Ideal Hydraulic Pressure Sensor/RConn1
  PS-S/LConn1 -- Ideal Hydraulic Pressure Sensor/RConn2

== system ssc_Probes_2014a_org/Magnetic/Flux ==
  Flux Sensor : fl_lib/Magnetic/Magnetic Sensors/Flux Sensor
      settings: SourceProductName=Simscape  SourceProductBaseCode=SS
  PS-S : nesl_utility/PS-Simulink Converter  PhysicalDomain=network_engine_domain  SubClassName=ps_output  LeftPortType=input  RightPortType=output  PseudoPeriodic=off  Frequencies=[]  Unit=Wb  AffineConversion=off
  Terminator : Terminator
  N : PMIOPort  Side=Left
  S : PMIOPort  Port=2  Side=Right
  wires:
  PS-S/1 -> [Flux]  "Flux"
  [Flux] -> Terminator/1
  connections:
  N/RConn1 -- Flux Sensor/LConn1
  Flux Sensor/RConn1 -- PS-S/LConn1
  S/RConn1 -- Flux Sensor/RConn2

== system ssc_Probes_2014a_org/Magnetic/MMF ==
  MMF Sensor : fl_lib/Magnetic/Magnetic Sensors/MMF Sensor
      settings: SourceProductName=Simscape  SourceProductBaseCode=SS
  Magnetic Reference : fl_lib/Magnetic/Magnetic Elements/Magnetic Reference  phi_Log=off  LocalVarNames=|phi  LocalVarDescs=|phi  LocalVarLogging=0
      settings: SourceProductName=Simscape  SourceProductBaseCode=SS
  PS-S : nesl_utility/PS-Simulink Converter  PhysicalDomain=network_engine_domain  SubClassName=ps_output  LeftPortType=input  RightPortType=output  PseudoPeriodic=off  Frequencies=[]  Unit=A  AffineConversion=off
  Terminator : Terminator
  N : PMIOPort  Side=Left
  wires:
  PS-S/1 -> [MMF]  "MMF"
  [MMF] -> Terminator/1
  connections:
  Magnetic Reference/LConn1 -- MMF Sensor/RConn2
  MMF Sensor/RConn1 -- PS-S/LConn1
  N/RConn1 -- MMF Sensor/LConn1

== system ssc_Probes_2014a_org/Magnetic/dMMF ==
  MMF Sensor : fl_lib/Magnetic/Magnetic Sensors/MMF Sensor
      settings: SourceProductName=Simscape  SourceProductBaseCode=SS
  PS-S : nesl_utility/PS-Simulink Converter  PhysicalDomain=network_engine_domain  SubClassName=ps_output  LeftPortType=input  RightPortType=output  PseudoPeriodic=off  Frequencies=[]  Unit=A  AffineConversion=off
  Terminator : Terminator
  N : PMIOPort  Side=Left
  S : PMIOPort  Port=2  Side=Right
  wires:
  PS-S/1 -> [dMMF]  "dMMF"
  [dMMF] -> Terminator/1
  connections:
  N/RConn1 -- MMF Sensor/LConn1
  MMF Sensor/RConn1 -- PS-S/LConn1
  S/RConn1 -- MMF Sensor/RConn2

== system ssc_Probes_2014a_org/Mechanical/AngVel ==
  Ideal Rotational Motion Sensor : fl_lib/Mechanical/Mechanical Sensors/Ideal Rotational Motion Sensor  offset=0 rad
  Mechanical Rotational Reference : fl_lib/Mechanical/Rotational Elements/Mechanical Rotational Reference  t_Log=off  LocalVarNames=|t  LocalVarDescs=|t  LocalVarLogging=0
  PS-S : nesl_utility/PS-Simulink Converter  PhysicalDomain=network_engine_domain  SubClassName=ps_output  LeftPortType=input  RightPortType=output  PseudoPeriodic=off  Frequencies=[]  Unit=rad/s  AffineConversion=off
  Terminator : Terminator
  R : PMIOPort  Side=Left
  wires:
  PS-S/1 -> [AngVel]  "AngVel"
  [AngVel] -> Terminator/1
  connections:
  Ideal Rotational Motion Sensor/RConn2 -- PS-S/LConn1
  Mechanical Rotational Reference/LConn1 -- Ideal Rotational Motion Sensor/RConn1
  R/RConn1 -- Ideal Rotational Motion Sensor/LConn1

== system ssc_Probes_2014a_org/Mechanical/Angle ==
  Ideal Rotational Motion Sensor : fl_lib/Mechanical/Mechanical Sensors/Ideal Rotational Motion Sensor  offset=0 rad
  Mechanical Rotational Reference : fl_lib/Mechanical/Rotational Elements/Mechanical Rotational Reference  t_Log=off  LocalVarNames=|t  LocalVarDescs=|t  LocalVarLogging=0
  PS-S : nesl_utility/PS-Simulink Converter  PhysicalDomain=network_engine_domain  SubClassName=ps_output  LeftPortType=input  RightPortType=output  PseudoPeriodic=off  Frequencies=[]  Unit=rad  AffineConversion=off
  Terminator : Terminator
  R : PMIOPort  Side=Left
  wires:
  PS-S/1 -> [Angle]  "Angle"
  [Angle] -> Terminator/1
  connections:
  R/RConn1 -- Ideal Rotational Motion Sensor/LConn1
  Mechanical Rotational Reference/LConn1 -- Ideal Rotational Motion Sensor/RConn1
  PS-S/LConn1 -- Ideal Rotational Motion Sensor/RConn3

== system ssc_Probes_2014a_org/Mechanical/Force ==
  Ideal Force Sensor : fl_lib/Mechanical/Mechanical Sensors/Ideal Force Sensor
  PS-S : nesl_utility/PS-Simulink Converter  PhysicalDomain=network_engine_domain  SubClassName=ps_output  LeftPortType=input  RightPortType=output  PseudoPeriodic=off  Frequencies=[]  Unit=N  AffineConversion=off
  Terminator : Terminator
  R : PMIOPort  Side=Left
  C : PMIOPort  Port=2  Side=Right
  wires:
  PS-S/1 -> [Force]  "Force"
  [Force] -> Terminator/1
  connections:
  C/RConn1 -- Ideal Force Sensor/RConn1
  Ideal Force Sensor/RConn2 -- PS-S/LConn1
  R/RConn1 -- Ideal Force Sensor/LConn1

== system ssc_Probes_2014a_org/Mechanical/Position ==
  Ideal Translational Motion Sensor : fl_lib/Mechanical/Mechanical Sensors/Ideal Translational Motion Sensor  offset=0 m
  Mechanical Translational Reference : fl_lib/Mechanical/Translational Elements/Mechanical Translational Reference  f_Log=off  LocalVarNames=|f  LocalVarDescs=|f  LocalVarLogging=0
  PS-S : nesl_utility/PS-Simulink Converter  PhysicalDomain=network_engine_domain  SubClassName=ps_output  LeftPortType=input  RightPortType=output  PseudoPeriodic=off  Frequencies=[]  Unit=m  AffineConversion=off
  Terminator : Terminator
  R : PMIOPort  Side=Left
  wires:
  PS-S/1 -> [Position]  "Position"
  [Position] -> Terminator/1
  connections:
  PS-S/LConn1 -- Ideal Translational Motion Sensor/RConn3
  Mechanical Translational Reference/LConn1 -- Ideal Translational Motion Sensor/RConn1
  R/RConn1 -- Ideal Translational Motion Sensor/LConn1

== system ssc_Probes_2014a_org/Mechanical/Torque ==
  Ideal Torque Sensor : fl_lib/Mechanical/Mechanical Sensors/Ideal Torque Sensor
  PS-S : nesl_utility/PS-Simulink Converter  PhysicalDomain=network_engine_domain  SubClassName=ps_output  LeftPortType=input  RightPortType=output  PseudoPeriodic=off  Frequencies=[]  Unit=N*m  AffineConversion=off
  Terminator : Terminator
  R : PMIOPort  Side=Left
  C : PMIOPort  Port=2  Side=Right
  wires:
  PS-S/1 -> [Torque]  "Torque"
  [Torque] -> Terminator/1
  connections:
  R/RConn1 -- Ideal Torque Sensor/LConn1
  Ideal Torque Sensor/RConn2 -- PS-S/LConn1
  C/RConn1 -- Ideal Torque Sensor/RConn1

== system ssc_Probes_2014a_org/Mechanical/Velocity ==
  Ideal Translational Motion Sensor : fl_lib/Mechanical/Mechanical Sensors/Ideal Translational Motion Sensor  offset=0 m
  Mechanical Translational Reference : fl_lib/Mechanical/Translational Elements/Mechanical Translational Reference  f_Log=off  LocalVarNames=|f  LocalVarDescs=|f  LocalVarLogging=0
  PS-S : nesl_utility/PS-Simulink Converter  PhysicalDomain=network_engine_domain  SubClassName=ps_output  LeftPortType=input  RightPortType=output  PseudoPeriodic=off  Frequencies=[]  Unit=m/s  AffineConversion=off
  Terminator : Terminator
  R : PMIOPort  Side=Left
  wires:
  PS-S/1 -> [Velocity]  "Velocity"
  [Velocity] -> Terminator/1
  connections:
  Ideal Translational Motion Sensor/RConn2 -- PS-S/LConn1
  R/RConn1 -- Ideal Translational Motion Sensor/LConn1
  Mechanical Translational Reference/LConn1 -- Ideal Translational Motion Sensor/RConn1

== system ssc_Probes_2014a_org/Mechanical/dAngVel ==
  Ideal Rotational Motion Sensor : fl_lib/Mechanical/Mechanical Sensors/Ideal Rotational Motion Sensor  offset=0 rad
  PS-S : nesl_utility/PS-Simulink Converter  PhysicalDomain=network_engine_domain  SubClassName=ps_output  LeftPortType=input  RightPortType=output  PseudoPeriodic=off  Frequencies=[]  Unit=rad/s  AffineConversion=off
  Terminator : Terminator
  R : PMIOPort  Side=Left
  C : PMIOPort  Port=2  Side=Right
  wires:
  PS-S/1 -> [dAngVel]  "dAngVel"
  [dAngVel] -> Terminator/1
  connections:
  R/RConn1 -- Ideal Rotational Motion Sensor/LConn1
  C/RConn1 -- Ideal Rotational Motion Sensor/RConn1
  Ideal Rotational Motion Sensor/RConn2 -- PS-S/LConn1

== system ssc_Probes_2014a_org/Mechanical/dAngle ==
  Ideal Rotational Motion Sensor : fl_lib/Mechanical/Mechanical Sensors/Ideal Rotational Motion Sensor  offset=0 rad
  PS-S : nesl_utility/PS-Simulink Converter  PhysicalDomain=network_engine_domain  SubClassName=ps_output  LeftPortType=input  RightPortType=output  PseudoPeriodic=off  Frequencies=[]  Unit=rad  AffineConversion=off
  Terminator : Terminator
  R : PMIOPort  Side=Left
  C : PMIOPort  Port=2  Side=Right
  wires:
  PS-S/1 -> [dAngle]  "dAngle"
  [dAngle] -> Terminator/1
  connections:
  PS-S/LConn1 -- Ideal Rotational Motion Sensor/RConn3
  C/RConn1 -- Ideal Rotational Motion Sensor/RConn1
  R/RConn1 -- Ideal Rotational Motion Sensor/LConn1

== system ssc_Probes_2014a_org/Mechanical/dPosition ==
  Ideal Translational Motion Sensor : fl_lib/Mechanical/Mechanical Sensors/Ideal Translational Motion Sensor  offset=0 m
  PS-S : nesl_utility/PS-Simulink Converter  PhysicalDomain=network_engine_domain  SubClassName=ps_output  LeftPortType=input  RightPortType=output  PseudoPeriodic=off  Frequencies=[]  Unit=m  AffineConversion=off
  Terminator : Terminator
  R : PMIOPort  Side=Left
  C : PMIOPort  Port=2  Side=Right
  wires:
  PS-S/1 -> [dPosition]  "dPosition"
  [dPosition] -> Terminator/1
  connections:
  R/RConn1 -- Ideal Translational Motion Sensor/LConn1
  C/RConn1 -- Ideal Translational Motion Sensor/RConn1
  PS-S/LConn1 -- Ideal Translational Motion Sensor/RConn3

== system ssc_Probes_2014a_org/Mechanical/dVelocity ==
  Ideal Translational Motion Sensor : fl_lib/Mechanical/Mechanical Sensors/Ideal Translational Motion Sensor  offset=0 m
  PS-S : nesl_utility/PS-Simulink Converter  PhysicalDomain=network_engine_domain  SubClassName=ps_output  LeftPortType=input  RightPortType=output  PseudoPeriodic=off  Frequencies=[]  Unit=m/s  AffineConversion=off
  Terminator : Terminator
  R : PMIOPort  Side=Left
  C : PMIOPort  Port=2  Side=Right
  wires:
  PS-S/1 -> [dVelocity]  "dVelocity"
  [dVelocity] -> Terminator/1
  connections:
  C/RConn1 -- Ideal Translational Motion Sensor/RConn1
  R/RConn1 -- Ideal Translational Motion Sensor/LConn1
  PS-S/LConn1 -- Ideal Translational Motion Sensor/RConn2

== system ssc_Probes_2014a_org/Pneumatic/AbsPressure ==
  PS-S : nesl_utility/PS-Simulink Converter  PhysicalDomain=network_engine_domain  SubClassName=ps_output  LeftPortType=input  RightPortType=output  PseudoPeriodic=off  Frequencies=[]  Unit=Pa  AffineConversion=off
  Pneumatic Absolute Reference : fl_lib/Pneumatic/Pneumatic Elements/Pneumatic Absolute Reference  G_Log=off  Q_Log=off  LocalVarNames=|G|Q  LocalVarDescs=|G|Q  LocalVarLogging=[0 0]
      settings: SourceProductName=Simscape  SourceProductBaseCode=SS
  Pneumatic Pressure & Temperature Sensor : fl_lib/Pneumatic/Pneumatic Sensors/Pneumatic Pressure & Temperature Sensor
      settings: SourceProductName=Simscape  SourceProductBaseCode=SS
  Terminator : Terminator
  A : PMIOPort  Side=Left
  wires:
  PS-S/1 -> [AbsPressure]  "AbsPressure"
  [AbsPressure] -> Terminator/1
  connections:
  A/RConn1 -- Pneumatic Pressure & Temperature Sensor/LConn1
  Pneumatic Absolute Reference/LConn1 -- Pneumatic Pressure & Temperature Sensor/RConn1
  PS-S/LConn1 -- Pneumatic Pressure & Temperature Sensor/RConn2
